simulink model "scheme_pos_control_yawcontrol"  (R2025a)
settings: Solver=ode3  StartTime=0.0  StopTime=40  FixedStep=dt  RelTol=1e-3
values from neighbouring files (symbols this model uses):
  dt = 0.0005    [Planning_Sim.m]
  goal_pos = waypoints(end, :)'    [Planning_Sim.m]
  initial_positions_rad = rawJointPositions(1, :)'    [manipulator_sim.m]
  manipulator_position_data = positions_final    [manipulator_sim.m]
  manipulator_time_vector = time_final    [manipulator_sim.m]
  map_scale = 0.5    [Planning_Sim.m]
  op_space_pose_trajectory = zeros(4, 4, num_points)    [Planning_Sim.m]
  waypoints = pathObj.States(:, 1:2)    [Planning_Sim.m]
  x0 = zeros(14, 1)    [Planning_Sim.m]
undefined symbols (not defined in the file or in its folder): control_params, p, X, Y, Z
libraries: sm_lib x179, nesl_utility x28, fl_lib x3
(part 5 of 5)

== matlab function scheme_pos_control_yawcontrol/BallBot Plant1/MATLAB Function ==
  data: dx output; x input; p parameter; tau input; wrench_ext input
function dx = stateDerivative3D_with_exforce(x, p, tau, wrench_ext)
    % MODIFICATION 1: The function now accepts a 4th argument, 'wrench_ext',
    % which is a vector containing the external forces and torques from Simulink.
    
    % Unpack state vector (10 elements)
    theta_x = x(1); dot_theta_x = x(6);
    theta_y = x(2); dot_theta_y = x(7);
    theta_z = x(3); dot_theta_z = x(8);
    % phi_x   = x(4); % Not needed for dynamics
    % phi_y   = x(5); % Not needed for dynamics
    dot_phi_x   = x(9);
    dot_phi_y   = x(10);
    
    % Unpack input torques
    tau_x = tau(1);
    tau_y = tau(2);
    tau_z = tau(3);

     % Unpack the external wrench vector from the new input ---
    % Expected order: [F_px, F_py, F_pz, tau_px, tau_py]
    F_px   = wrench_ext(1);
    F_py   = wrench_ext(2);
    F_pz   = wrench_ext(3);
    tau_px = wrench_ext(4);
    tau_py = wrench_ext(5);

    % --- Prepare arguments for auto-generated functions ---
    % Create separate parameter vectors for each plane, now including h_app
    % Note: I_Ux is for roll, I_Uy is for pitch.
    params_arg_roll = [p.m_U,  p.I_Uy, p.I_Ux, p.l_U, p.m_S, p.I_S, p.r_S, p.g, p.h_app, p.b_theta, p.b_phi];
    params_arg_pitch = [p.m_U, p.I_Uy, p.I_Ux, p.l_U, p.m_S, p.I_S, p.r_S, p.g,p.h_app, p.b_theta, p.b_phi];
    
    external_vars_x = [F_py, F_pz, tau_px]; % For Roll dynamics
    external_vars_y = [F_px, F_pz, tau_py]; % For Pitch dynamics

    % --- X-Z Plane (Roll) Dynamics ---
    states_arg_x = [theta_x, dot_theta_x, dot_phi_x];
    inputs_arg_x = [tau_x];
    ddot_theta_x = copy_autogen_ddot_theta_x(states_arg_x, inputs_arg_x, params_arg_roll, external_vars_x);
    ddot_phi_x   = copy_autogen_ddot_phi_x(states_arg_x, inputs_arg_x, params_arg_roll, external_vars_x);
    

    % --- Y-Z Plane (Pitch) Dynamics ---
    states_arg_y = [theta_y, dot_theta_y, dot_phi_y];
    inputs_arg_y = [tau_y];
    ddot_theta_y = copy_autogen_ddot_theta_y(states_arg_y, inputs_arg_y, params_arg_pitch, external_vars_y);
    ddot_phi_y   = copy_autogen_ddot_phi_y(states_arg_y, inputs_arg_y, params_arg_pitch, external_vars_y);
    
    % --- Transversal Plane Dynamics (Yaw) ---
    % external forces at the center of the top surface are assumed not to produce yaw torque.
    ddot_theta_z = (tau_z - p.fz * dot_theta_z) / p.Iz;
    
    % --- Assemble the state derivative vector dx ---
    dx = [
        dot_theta_x;    % dx(1) = d(theta_x)/dt
        dot_theta_y;    % dx(2) = d(theta_y)/dt
        dot_theta_z;    % dx(3) = d(theta_z)/dt
        dot_phi_x;      % dx(4) = d(phi_x)/dt
        dot_phi_y;      % dx(5) = d(phi_y)/dt
        ddot_theta_x;   % dx(6) = d(dot_theta_x)/dt
        ddot_theta_y;   % dx(7) = d(dot_theta_y)/dt
        ddot_theta_z;   % dx(8) = d(dot_theta_z)/dt
        ddot_phi_x;     % dx(9) = d(dot_phi_x)/dt
        ddot_phi_y;     % dx(10)= d(dot_phi_y)/dt
    ];
end

== matlab function scheme_pos_control_yawcontrol/MATLAB Function ==
  settings: updateMethod=DISCRETE
  data: x input; phi_dot_c output; waypoints input; p parameter; simtime input; control_params parameter; is_final_segment output; dt parameter; position_error output
function [phi_dot_c,is_final_segment,position_error] = generate_ff_fb_velocity_command(x, waypoints, p, simtime, control_params,dt)
% =========================================================================
% ADVANCED FEEDFORWARD + FEEDBACK VELOCITY COMMAND GENERATOR
%
% Version: 5.0 - Hybrid Control for Final Approach
%
% This version uses the advanced path-following controller for the main
% trajectory and switches to a simple proportional position controller
% for the final segment to ensure stable regulation at the goal.
% =========================================================================

% --- Parametri ---
persistent processed_path;
persistent previous_waypoints;
persistent integral_pos_error; % NEW: Persistent variable for the integral term
v_max       = 0.3;
a_max       = 0.08;
Kp_feedback = 0.20; % Gain for path following on intermediate segments
lookahead_distance = 0.0;

% NEW: Proportional gain specifically for the final approach/regulation.
% You can tune this gain to get the desired stopping behavior.
Kp_final_approach = control_params.Kp;
Ki_final_approach = control_params.Ki; % Get the new Ki gain from your main script
% --- Stato attuale del robot ---
p_current = [p.r_S * x(5); -p.r_S * x(4)];
v_current = [p.r_S * x(2); -p.r_S * x(3)];

% --- Logica di Inizializzazione e Replanning (invariata) ---
if isempty(previous_waypoints)
    disp('First run: Initializing and processing path...');
    processed_path = preprocess_waypoints_with_blending(waypoints, v_max, a_max, ...
                                                        p_current, v_current, simtime);
    previous_waypoints = waypoints;
else
    if ~isequal(waypoints, previous_waypoints)
        disp('Waypoints changed: Replanning path from current state...');
        processed_path = preprocess_waypoints_with_blending(waypoints, v_max, a_max, ...
                                                            p_current, v_current, simtime);
        previous_waypoints = waypoints;
    end
end

% NEW: Initialize the integral term on the first run
if isempty(integral_pos_error)
    integral_pos_error = zeros(2,1);
end

% --- MODIFIED: HYBRID CONTROL LOGIC ---

% Get the current trajectory information, including the segment index
[v_ref_normal, current_segment, segment_is_valid, current_segment_idx] = get_reference_and_segment(processed_path, simtime);
num_total_segments = length(processed_path.segments);

% Check if we are on the final segment of the path.
is_final_segment = (segment_is_valid && current_segment_idx == num_total_segments);

if is_final_segment
    % --- FINAL APPROACH: PI Regulation Controller ---
    
    p_goal = waypoints(end, :)'; % The final destination
    position_error = p_goal - p_current;
    
    integral_pos_error = integral_pos_error + position_error * dt;
    % The velocity command is purely proportional to the position error.
    % NEW: The velocity command now has a Proportional and an Integral term
    v_cmd = Kp_final_approach * position_error + Ki_final_approach * integral_pos_error;
    
else
    % --- PATH FOLLOWING: Advanced Controller for Intermediate Segments ---
    % NEW: Reset the integral term when not in regulation mode.
    % This is crucial to prevent "integral wind-up".
    integral_pos_error = zeros(2,1);
    % This is the original advanced logic
    if segment_is_valid
        vec_start_to_robot = p_current - current_segment.p_start;
        projection_dist = dot(vec_start_to_robot, current_segment.direction);
        p_closest = current_segment.p_start + projection_dist * current_segment.direction;
        p_lookahead = p_closest + lookahead_distance * current_segment.direction;
        vec_start_to_lookahead = p_lookahead - current_segment.p_start;
        dist_start_to_lookahead = dot(vec_start_to_lookahead, current_segment.direction);
        if dist_start_to_lookahead > current_segment.distance
            p_target_for_feedback = current_segment.p_end;
        else
            p_target_for_feedback = p_lookahead;
        end
    else
        p_target_for_feedback = p_current; 
    end
    
    position_error = p_target_for_feedback - p_current;
    v_feedback = Kp_feedback * position_error;
    
    % Combine feedforward (from trapezoidal profile) and feedback
    v_cmd = v_ref_normal + v_feedback;
end

% --- Override for initialization phase (remains the same) ---
initialization_time = 3.0;
if simtime < initialization_time
    position_error_init = [0;0] - p_current;
    v_cmd = Kp_final_approach * position_error_init; % Use the regulation controller to hold at zero
end

% --- Final command generation (acts on v_cmd from either logic branch) ---
v_cmd_magnitude = norm(v_cmd);
if v_cmd_magnitude > v_max
    v_cmd = v_cmd / v_cmd_magnitude * v_max;
end
phi_dot_c = [v_cmd(1) / p.r_S; -v_cmd(2) / p.r_S];

end

% =========================================================================
% --- LOCAL HELPER FUNCTIONS ---
% =========================================================================
function processed_path = preprocess_waypoints_with_blending(waypoints, v_max, a_max, p_start_robot, v_start_robot, time_start_robot)
    effective_waypoints = [p_start_robot'; waypoints];
    num_waypoints = size(effective_waypoints, 1);
    num_segments = num_waypoints - 1;
    
    % --- Calcolo della geometria (invariato) ---
    segment_template = struct('p_start', zeros(2,1), 'p_end', zeros(2,1), 'distance', 0, 'direction', zeros(2,1));
    path_geom.segments = repmat(segment_template, 1, num_segments);
    for i = 1:num_segments
        p_start = effective_waypoints(i, :)';
        p_end   = effective_waypoints(i+1, :)';
        vec     = p_end - p_start;
        dist    = norm(vec);
        path_geom.segments(i).p_start   = p_start;
        path_geom.segments(i).p_end     = p_end;
        path_geom.segments(i).distance  = dist;
        if dist > 1e-6
            path_geom.segments(i).direction = vec / dist;
        else
            path_geom.segments(i).direction = zeros(2,1);
        end
    end
    
    % --- Calcolo delle velocità di transizione ---
    v_transitions = zeros(2, num_waypoints);
    v_transitions(:, 1) = v_start_robot;
    v_transitions(:, end) = [0; 0];
    alpha = 3.0;
    
    % MODIFIED: Corrected loop range to include the penultimate waypoint
    for i = 2:num_waypoints-1
        v_max_for_corner = v_max;
        % MODIFIED: Slow down for the corners leading into the last TWO segments
        if i >= num_waypoints - 2 
            v_max_for_corner = v_max / 2;
        end
        
        dir_in  = path_geom.segments(i-1).direction;
        dir_out = path_geom.segments(i).direction;
        cos_theta = dot(dir_in, dir_out);
        v_mag = v_max_for_corner * ((1 + cos_theta) / 2)^alpha;
        v_dir_vec = dir_in + dir_out;
        if norm(v_dir_vec) > 1e-6
            v_dir_normalized = v_dir_vec / norm(v_dir_vec);
        else
            v_dir_normalized = zeros(2,1);
            v_mag = 0;
        end
        v_transitions(:, i) = v_mag * v_dir_normalized;
    end
    
    % --- Calcolo del profilo trapezoidale per ogni segmento ---
    profile_template = struct('v_start',0,'v_cruise',0,'v_end',0,'t_accel',0,'t_const',0,'t_decel',0,'total_time',0,'start_time',0,'a_max',0);
    processed_segment_template = struct('profile',profile_template,'direction',zeros(2,1),'p_start',zeros(2,1),'p_end',zeros(2,1),'distance',0);
    processed_segments = repmat(processed_segment_template, 1, num_segments);
    
    cumulative_time = time_start_robot;
    for i = 1:num_segments
        % MODIFIED: Set v_max and a_max for the last TWO segments
        v_max_current = v_max;
        a_max_current = a_max;
        if i >= num_segments - 1 && num_segments > 1 % Check if it's one of the last two segments
            v_max_current = v_max / 3;
            a_max_current = a_max / 3;
        elseif num_segments == 1 % Handle the case of a single-segment path
             v_max_current = v_max / 2;
             a_max_current = a_max / 2;
        end

        segment = path_geom.segments(i);
        v_start = dot(v_transitions(:, i),   segment.direction);
        v_end   = dot(v_transitions(:, i+1), segment.direction);
        v_start = max(0, v_start);
        v_end   = max(0, v_end);
        
        dist_accel = (v_max_current^2 - v_start^2) / (2 * a_max_current);
        dist_decel = (v_max_current^2 - v_end^2)   / (2 * a_max_current);

        if (dist_accel + dist_decel) >= segment.distance
            v_peak_sq = (2*a_max_current*segment.distance + v_start^2 + v_end^2) / 2;
            v_cruise = sqrt(max(0, v_peak_sq));
            t_accel = (v_cruise - v_start) / a_max_current;
            t_const = 0;
            t_decel = (v_cruise - v_end) / a_max_current;
        else
            v_cruise = v_max_current;
            dist_const = segment.distance - dist_accel - dist_decel;
            t_accel = (v_cruise - v_start) / a_max_current;
            t_const = dist_const / v_cruise;
            t_decel = (v_cruise - v_end) / a_max_current;
        end
        
        processed_segments(i).profile.v_start  = v_start;
        processed_segments(i).profile.v_cruise = v_cruise;
        processed_segments(i).profile.v_end    = v_end;
        processed_segments(i).profile.t_accel  = max(0, t_accel);
        processed_segments(i).profile.t_const  = max(0, t_const);
        processed_segments(i).profile.t_decel  = max(0, t_decel);
        processed_segments(i).profile.total_time = processed_segments(i).profile.t_accel + processed_segments(i).profile.t_const + processed_segments(i).profile.t_decel;
        processed_segments(i).profile.start_time = cumulative_time;
        processed_segments(i).profile.a_max = a_max_current;
        
        processed_segments(i).direction = segment.direction;
        processed_segments(i).p_start = segment.p_start;
        processed_segments(i).p_end = segment.p_end;
        processed_segments(i).distance = segment.distance;
        
        cumulative_time = cumulative_time + processed_segments(i).profile.total_time;
    end
    processed_path.segments = processed_segments;
    processed_path.total_duration = cumulative_time;
end
% MODIFIED: Returns a fixed-size struct and a validity flag.
function [v_ref, segment, is_valid, current_segment_idx] = get_reference_and_segment(processed_path, simtime)
    % 1. Define templates
    profile_template = struct(...
        'v_start', 0, 'v_cruise', 0, 'v_end', 0, ...
        't_accel', 0, 't_const', 0, 't_decel', 0, ...
        'total_time', 0, 'start_time', 0, 'a_max', 0);
        
    segment_template = struct(...
        'profile', profile_template, 'direction', zeros(2,1), ...
        'p_start', zeros(2,1), 'p_end', zeros(2,1), 'distance', 0);
    
    % 2. Initialize outputs
    segment = segment_template; 
    v_ref = [0;0];
    is_valid = false;
    
    % FIX: Initialize the new output variable to a default value.
    % This ensures it is always defined, even if the 'if' block is skipped.
    current_segment_idx = 0; 
    
    % 3. Main Logic (This part is unchanged and correct)
    if ~isempty(processed_path) && ~isempty(processed_path.segments)
        % This loop finds the correct segment index and overwrites the default '0'
        for i = 1:length(processed_path.segments)
            if simtime >= processed_path.segments(i).profile.start_time
                current_segment_idx = i;
            else
                break;
            end
        end
        segment = processed_path.segments(current_segment_idx);
        is_valid = true;
        prof = segment.profile;
        
        a_max_current = prof.a_max; 
        
        if simtime >= processed_path.total_duration
            v_ref = [0; 0];
            return;
        end
        time_in_segment = simtime - prof.start_time;
        current_speed = 0.0;
        
        if time_in_segment < prof.t_accel
            current_speed = prof.v_start + a_max_current * time_in_segment;
        elseif time_in_segment < (prof.t_accel + prof.t_const)
            current_speed = prof.v_cruise;
        else
            time_in_decel = time_in_segment - (prof.t_accel + prof.t_const);
            current_speed = prof.v_cruise - a_max_current * time_in_decel;
        end
        v_ref = max(0, current_speed) * segment.direction;
    end
end

== matlab function scheme_pos_control_yawcontrol/MATLAB Function1 ==
  settings: updateMethod=DISCRETE
  data: alpha_traj input; thetaz_des output; thetaz input; external_wrench input
function thetaz_des = calculate_desired_yaw(alpha_traj, thetaz, external_wrench)
% =========================================================================
% CALCULATE DESIRED YAW (v3.0 - With Continuous Unwrapping)
%
% This version removes the final normalization and implements an unwrapping
% algorithm. This allows the desired yaw angle to grow continuously beyond
% +/- 180 degrees, enabling smooth, continuous rotation without wrapping.
% =========================================================================

    % --- NEW: Persistent variable to store the last output for unwrapping ---
    persistent thetaz_des_old;
    if isempty(thetaz_des_old)
        % Initialize to the robot's starting yaw angle on the first run
        thetaz_des_old = thetaz;
    end

    % --- Step 1 & 2: Calculate instantaneous desired angle (Unchanged) ---
    F_dist_world_x = external_wrench(1);
    F_dist_world_y = external_wrench(2);
    local_psi_des = 0.0;
    force_magnitude = sqrt(F_dist_world_x^2 + F_dist_world_y^2);
    
    if force_magnitude < 1e-6
        local_psi_des = alpha_traj;
    else
        c = cos(-thetaz);
        s = sin(-thetaz);
        F_dist_body_x = c * F_dist_world_x - s * F_dist_world_y;
        F_dist_body_y = s * F_dist_world_x + c * F_dist_world_y;
        beta_dist_body = atan2(F_dist_body_y, F_dist_body_x);
        local_psi_des = alpha_traj - beta_dist_body;
    end
    
    % --- Step 3: UNWRAP the angle for continuous rotation ---
    % Instead of normalizing the final value, we normalize the DIFFERENCE
    % between the new instantaneous angle and the last continuous angle.
    
    angle_diff = local_psi_des - thetaz_des_old;
    
    % Find the shortest rotation path (wrap the difference to [-pi, pi])
    angle_diff_wrapped = atan2(sin(angle_diff), cos(angle_diff));
    
    % Add this shortest-path difference to the previous angle to get the
    % new continuous, unwrapped angle.
    thetaz_des = thetaz_des_old + angle_diff_wrapped;
    
    % --- Step 4: Update the persistent variable for the next time step ---
    thetaz_des_old = thetaz_des;

end
